simulink model "PWM_signal_and_complement_signal_generator"  (R2024b)
settings: Solver=VariableStepAuto  StartTime=0.0  StopTime=0.05  RelTol=1e-3
libraries: spsSawtoothGeneratorLib x1
settings Model: Creator=User  LastModifiedBy=User

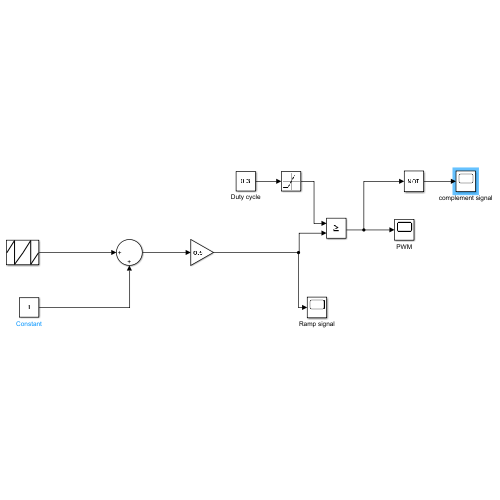
[thumbnail: Simulink's stored preview of the top-level diagram]
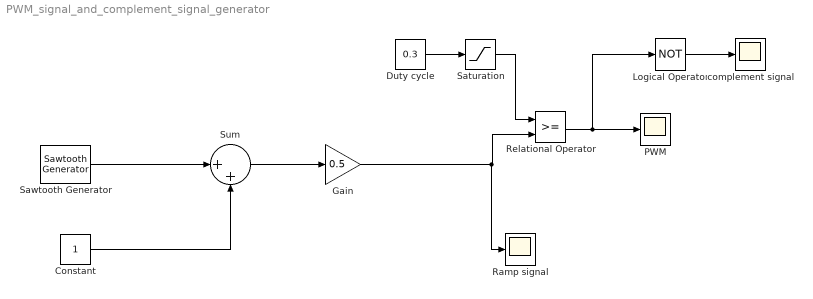
== system PWM_signal_and_complement_signal_generator ==
  Constant : Constant
  Duty cycle : Constant  Value=0.3
  Gain : Gain  Gain=0.5
  Logical Operator : Logic  Operator=NOT  AllPortsSameDT=off  OutDataTypeStr=boolean
  PWM : Scope
  Ramp signal : Scope
  Relational Operator : RelationalOperator  OutDataTypeStr=boolean  RndMeth=Simplest  InputSameDT=off
  Saturation : Saturate  UpperLimit=1  LowerLimit=0
  Sawtooth Generator : spsSawtoothGeneratorLib/Sawtooth Generator  Freq=20e3  Phase=180  Ts=0
  Sum : Sum  Inputs=|++
  complement signal : Scope
  wires:
  Sawtooth Generator/1 -> Sum/1
  Constant/1 -> Sum/2
  Sum/1 -> Gain/1
  Gain/1 -> Ramp signal/1, Relational Operator/2
  Relational Operator/1 -> Logical Operator/1, PWM/1
  Duty cycle/1 -> Saturation/1
  Saturation/1 -> Relational Operator/1
  Logical Operator/1 -> complement signal/1
